simulink model "Simple_RC_Circuit"  (R2019a)
settings: Solver=VariableStepAuto  StartTime=0.0  StopTime=10.0  RelTol=1e-3
undefined symbols (not defined in the file or in its folder): C, R
settings Model: Creator=T.S  LastModifiedBy=T.S

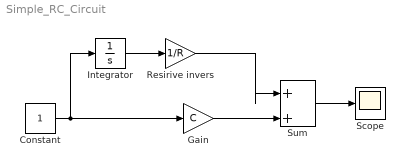
== system Simple_RC_Circuit ==
  Constant : Constant
  Gain : Gain  Gain=C
  Integrator : Integrator
  Resirive invers : Gain  Gain=1/R
  Scope : Scope
  Sum : Sum  Inputs=|++
  wires:
  Sum/1 -> Scope/1
  Constant/1 -> Integrator/1, Gain/1
  Gain/1 -> Sum/2
  Resirive invers/1 -> Sum/1
  Integrator/1 -> Resirive invers/1
